simulink model "assignment7newmodel"  (R2015a)
settings: Solver=ode45  StartTime=0.0  StopTime=168  RelTol=1e-3
PreLoadFcn:
  | assign7new
values from neighbouring files (symbols this model uses):
  c = 1005.4    [assign7new.m]
  cost = .19    (= 0.19)    [assign7new.m]
  M = volumeHouse*airDensity    [assign7new.m]
  Mdot = flowrate*3600    (= 1800)    [assign7new.m]
  Req = Rtot/(totalareaWalls+totalareawindr+roofArea)    [assign7new.m]
  THeater = 40    [assign7new.m]
  TinIC = 20    [assign7new.m]
settings Model: Creator=kate  LastModifiedBy=kate
settings DataIOCC: ExternalInput=[time, Weekly]  LoadExternalInput=on

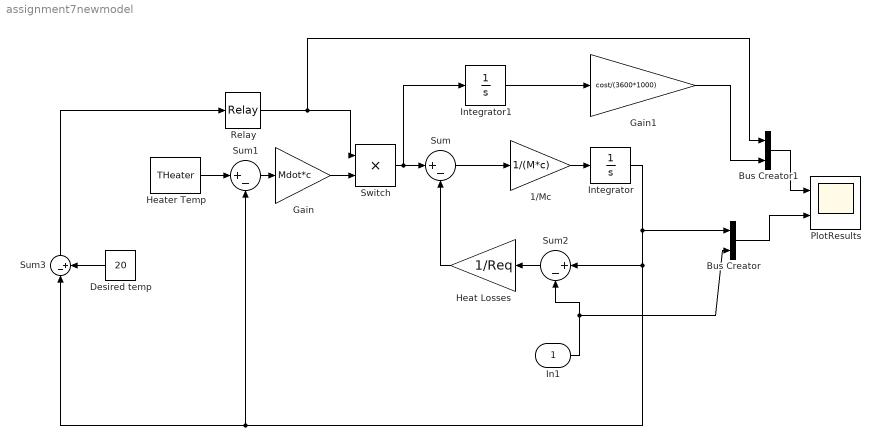
== system assignment7newmodel ==
  In1 : Inport
  "1/Mc " : Gain  Gain=1/(M*c)
  Bus Creator : BusCreator  Inputs=2
  Bus Creator1 : BusCreator  Inputs=2
  Desired temp : Constant  Value=20
  Gain : Gain  Gain=Mdot*c
  Gain1 : Gain  Gain=cost/(3600*1000)
  Heat Losses : Gain  Gain=1/Req
  "Heater Temp " : Constant  Value=THeater
  Integrator : Integrator  InitialCondition=TinIC
  Integrator1 : Integrator
  PlotResults : Scope  NumInputPorts=2
      settings: TimeRange=50  YMin=0.2~9.58  YMax=2~9.75  SaveName=a
  Relay : Relay  OnSwitchValue=1.5  OffSwitchValue=-1.5
  Sum : Sum  Inputs=|+-
  Sum1 : Sum  Inputs=|+-
  Sum2 : Sum  Inputs=|+-
  Sum3 : Sum  Inputs=|-+
  Switch : Product
  wires:
  "1/Mc "/1 -> Integrator/1
  "Heater Temp "/1 -> Sum1/1
  Sum1/1 -> Gain/1
  Sum/1 -> "1/Mc "/1
  Sum2/1 -> Heat Losses/1
  Heat Losses/1 -> Sum/2
  Desired temp/1 -> Sum3/2
  Switch/1 -> Integrator1/1, Sum/1
  Gain/1 -> Switch/2
  Sum3/1 -> Relay/1
  Relay/1 -> Bus Creator1/1, Switch/1
  Integrator1/1 -> Gain1/1
  Integrator/1 -> Bus Creator/1, Sum3/1, Sum1/2, Sum2/1
  In1/1 -> Bus Creator/2, Sum2/2
  Bus Creator/1 -> PlotResults/2
  Bus Creator1/1 -> PlotResults/1
  Gain1/1 -> Bus Creator1/2
